simulink model "modSFunc_test_zeros"  (R2024b)
settings: Solver=ode4  StartTime=0.0  StopTime=TMax  FixedStep=DT  MaxStep=DT  RelTol=1e-3  EnableMultiTasking=on
settings Model: Creator=bjonkman  LastModifiedBy=mcdevin
settings SolverCC: AlgebraicLoopSolver=TrustRegion
settings DataIOCC: LimitDataPoints=on  SaveFormat=Array  SignalLoggingSaveFormat=ModelDataLogs  SaveOutput=off  SaveTime=off  ReturnWorkspaceOutputs=off  SignalLoggingName=sigsOut
settings OptimizationCC: ExpressionDepthLimit=2147483647  LifeSpan=inf
settings DebuggingCC: SaveWithParameterizedLinksMsg=none  UnderspecifiedInitializationDetection=Classic  MergeDetectMultiDrivingBlocksExec=none  SignalResolutionControl=TryResolveAllWithWarning  MultiTaskDSMMsg=warning  MultiTaskCondExecSysMsg=none  FcnCallInpInsideContextMsg=warning  UnconnectedInputMsg=warning  UnconnectedOutputMsg=warning  UnconnectedLineMsg=warning  StateNameClashWarn=warning  SFUnexpectedBacktrackingDiag=warning  SFNoUnconditionalDefaultTransitionDiag=warning  SFExecutionAtInitializationDiag=none  ArithmeticOperatorsInVariantConditions=warning
settings HardwareCC: ProdBitPerPointer=32  ProdBitPerSizeT=32  ProdBitPerPtrDiffT=32  ProdLargestAtomicFloat=None  ProdIntDivRoundTo=Undefined  ProdEndianess=Unspecified  ProdWordSize=32  ProdHWDeviceType=32-bit Generic  TargetUnknown=on
settings ModelReferenceCC: EnableRefExpFcnMdlSchedulingChecks=on  PropagateSignalLabelsOutOfModel=off
settings SFSimCC: SimUseLocalCustomCode=off  CustomCodeUndefinedFunction=UseInterfaceOnly
settings RTWCC: RTWUseLocalCustomCode=off  GPUComputeCapability=3.5  DLArmComputeVersion=19.05
settings CodeAppCC: StateflowObjectComments=on
settings GRTTargetCC: TargetLangStandard=C89/C90 (ANSI)  CombineOutputUpdateFcns=off  GRTInterface=on
settings ConfigComp: CovMetricSettings=dw  CovSaveCumulativeToWorkspaceVar=on  CovSaveSingleToWorkspaceVar=on  CovExternalEMLEnable=off

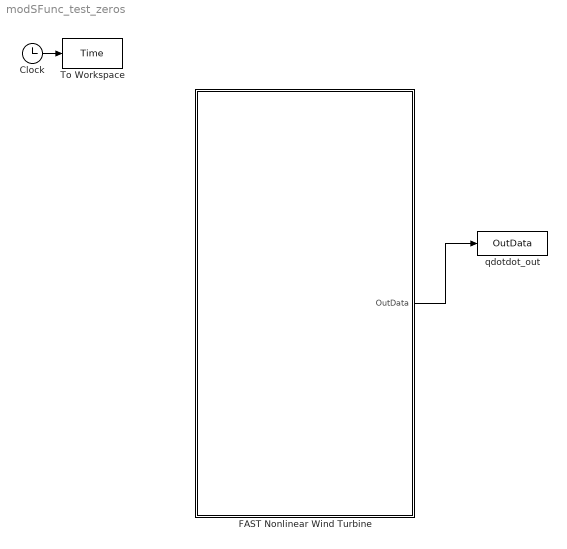
== system modSFunc_test_zeros ==
  Clock : Clock
  FAST Nonlinear Wind Turbine : Subsystem  mask(FAST Nonlinear Wind Turbine){}
      mask help: This block contains the FAST S-Function.
      mask init:
      | clear FAST_SFunc
  To Workspace : ToWorkspace  VariableName=Time  SampleTime=-1
  qdotdot_out : ToWorkspace  VariableName=OutData  SampleTime=-1
  wires:
  Clock/1 -> To Workspace/1
  FAST Nonlinear Wind Turbine/1(OutData) -> qdotdot_out/1

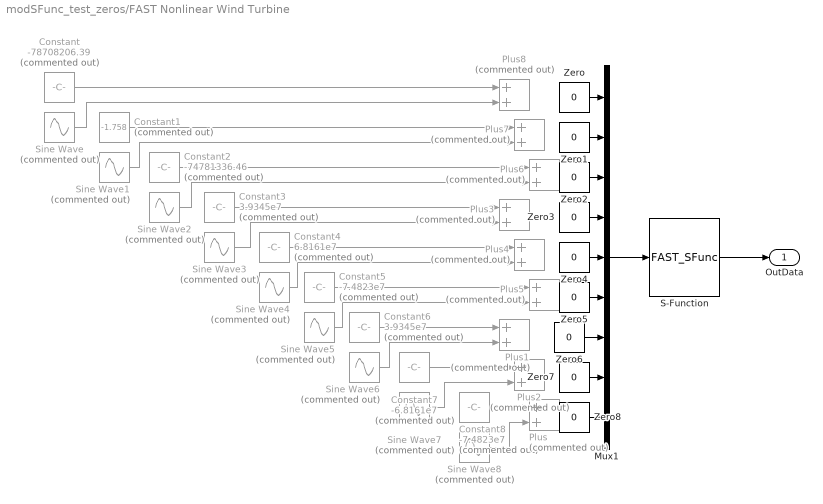
== system modSFunc_test_zeros/FAST Nonlinear Wind Turbine ==
  Constant : Constant  Commented=on  Value=-78708206.39
  Constant1 : Constant  Commented=on  Value=-1.758
  Constant2 : Constant  Commented=on  Value=-74781336.46
  Constant3 : Constant  Commented=on  Value=3.9345e7
  Constant4 : Constant  Commented=on  Value=6.8161e7
  Constant5 : Constant  Commented=on  Value=-7.4823e7
  Constant6 : Constant  Commented=on  Value=3.9345e7
  Constant7 : Constant  Commented=on  Value=-6.8161e7
  Constant8 : Constant  Commented=on  Value=-7.4823e7
  Mux1 : Mux  Inputs=9
  Plus{,1..8} (9 alike) : Sum  Commented=on
  S-Function : S-Function  FunctionName=FAST_SFunc  Parameters=FAST_InputFileName, TMax, 0  SFunctionDeploymentMode=off  EnableBusSupport=off
  Sine Wave : Sin  Commented=on  Amplitude=22011  SampleTime=0
  Sine Wave1 : Sin  Commented=on  Amplitude=510.6  SampleTime=0
  Sine Wave2 : Sin  Commented=on  Amplitude=35425  SampleTime=0
  Sine Wave3 : Sin  Commented=on  Amplitude=25362  SampleTime=0
  Sine Wave4 : Sin  Commented=on  Amplitude=4632  SampleTime=0
  Sine Wave5 : Sin  Commented=on  Amplitude=28207  SampleTime=0
  Sine Wave6 : Sin  Commented=on  Amplitude=24550  SampleTime=0
  Sine Wave7 : Sin  Commented=on  Amplitude=5087  SampleTime=0
  Sine Wave8 : Sin  Commented=on  Amplitude=28166  SampleTime=0
  Zero{,1..8} (9 alike) : Constant  Value=0  OutDataTypeStr=Inherit: Inherit via back propagation
  OutData : Outport
  wires:
  S-Function/1 -> OutData/1
  Mux1/1 -> S-Function/1
  Constant8/1 -> Plus/1
  Sine Wave8/1 -> Plus/2
  Constant7/1 -> Plus2/1
  Sine Wave7/1 -> Plus2/2
  Constant6/1 -> Plus1/1
  Sine Wave6/1 -> Plus1/2
  Constant5/1 -> Plus5/1
  Sine Wave5/1 -> Plus5/2
  Constant4/1 -> Plus4/1
  Sine Wave4/1 -> Plus4/2
  Constant3/1 -> Plus3/1
  Sine Wave3/1 -> Plus3/2
  Constant2/1 -> Plus6/1
  Sine Wave2/1 -> Plus6/2
  Constant1/1 -> Plus7/1
  Sine Wave1/1 -> Plus7/2
  Sine Wave/1 -> Plus8/2
  Constant/1 -> Plus8/1
  Zero/1 -> Mux1/1
  Zero8/1 -> Mux1/9
  Zero7/1 -> Mux1/8
  Zero6/1 -> Mux1/7
  Zero5/1 -> Mux1/6
  Zero4/1 -> Mux1/5
  Zero3/1 -> Mux1/4
  Zero2/1 -> Mux1/3
  Zero1/1 -> Mux1/2
